simulink model "air_speed_control"  (R2016a)
settings: Solver=VariableStepAuto  StartTime=0.0  StopTime=10.0  RelTol=1e-6
model workspace (MAT data in the model file):
  A1 = 0.00125663706144
  A2 = 0.00105557513161
  L = 0.3
  M_huosai = 20
  P0 = 101300
  R = 287.1
  T1 = 293
  T2 = 293
  Ts = 293
  k = 1.4
undefined symbols (not defined in the file or in its folder): vd
settings Model: Creator=xlh  LastModifiedBy=xlh

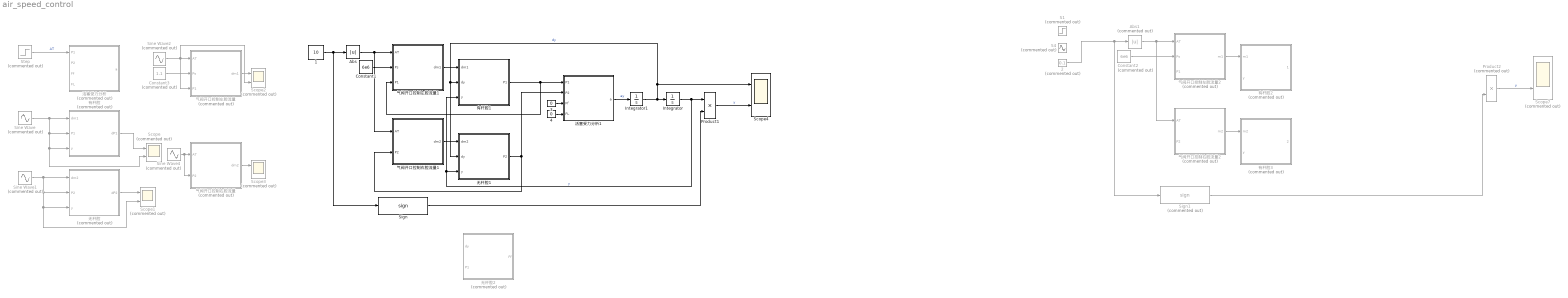
== system air_speed_control ==
  1 : Constant  Value=10
  2 : Constant  Commented=on  Value=0.1
  3 : Constant  Value=0
  4 : Constant  Value=0
  Abs : Abs
  Abs1 : Abs  Commented=on
  Constant1 : Constant  Value=6e6
  Constant2 : Constant  Commented=on  Value=6e6
  Constant3 : Constant  Commented=on  Value=1.1
  Integrator : Integrator
  Integrator1 : Integrator
  Product1 : Product
  Product2 : Product  Commented=on
  S1 : Step  Commented=on  SampleTime=0
  S4 : Sin  Commented=on  SampleTime=0
  Scope{,1..3,7} (5 alike) : Scope  Commented=on  NumInputPorts=2
  Scope4 : Scope  NumInputPorts=2
  Sign : Signum
  Sign1 : Signum  Commented=on
  Sine Wave{,1..2,4} (4 alike) : Sin  Commented=on  SampleTime=0
  Step : Step  Commented=on  SampleTime=0
  无杆腔 : Subsystem  Commented=on
  无杆腔1 : Subsystem
  无杆腔2 : Subsystem  Commented=on
  有杆腔 : Subsystem  Commented=on
  有杆腔1 : Subsystem
  有杆腔2 : Subsystem  Commented=on
  有杆腔3 : Subsystem  Commented=on
  气阀开口控制右腔流量 : Subsystem  Commented=on
  气阀开口控制右腔流量1 : Subsystem
  气阀开口控制右腔流量2 : Subsystem  Commented=on
  气阀开口控制左腔流量 : Subsystem  Commented=on
  气阀开口控制左腔流量1 : Subsystem
  气阀开口控制左腔流量2 : Subsystem  Commented=on
  活塞受力分析 : Subsystem  Commented=on
  活塞受力分析1 : Subsystem
  wires:
  Step/1 -> 活塞受力分析/1(P1)  "AT"
  Sine Wave/1 -> Scope/2, 有杆腔/3(y), 有杆腔/2(P1), 有杆腔/1(dm1)
  有杆腔/1(dP1) -> Scope/1
  Sine Wave1/1 -> Scope1/2, 无杆腔/3(y), 无杆腔/2(P2), 无杆腔/1(dm2)
  无杆腔/1(dP2) -> Scope1/1
  Constant3/1 -> 气阀开口控制左腔流量/2(Ps)
  Sine Wave2/1 -> 气阀开口控制左腔流量/3(P1), Scope2/2, 气阀开口控制左腔流量/1(AT)
  气阀开口控制左腔流量/1(dm1) -> Scope2/1
  Sine Wave4/1 -> 气阀开口控制右腔流量/2(P2), 气阀开口控制右腔流量/1(AT)
  气阀开口控制右腔流量/1(dm2) -> Scope3/1
  气阀开口控制左腔流量1/1(dm1) -> 有杆腔1/1(dm1)
  有杆腔1/1(P1) -> 气阀开口控制左腔流量1/3(P1), 活塞受力分析1/1(P1)
  活塞受力分析1/1(a) -> Integrator1/1  "ay"
  Integrator1/1 -> Integrator/1, 有杆腔1/2(dy), 无杆腔1/2(dy), Scope4/1  "dy"
  Constant1/1 -> 气阀开口控制左腔流量1/2(Ps)
  气阀开口控制右腔流量1/1(dm2) -> 无杆腔1/1(dm2)
  4/1 -> 活塞受力分析1/4(FL)
  无杆腔1/1(P2) -> 活塞受力分析1/2(P2), 气阀开口控制右腔流量1/2(P2)
  Integrator/1 -> 无杆腔1/3(y), 有杆腔1/3(y), Product1/1  "y"
  Product1/1 -> Scope4/2  "y"
  Sign/1 -> Product1/2
  1/1 -> Abs/1, Sign/1
  Abs/1 -> 气阀开口控制右腔流量1/1(AT), 气阀开口控制左腔流量1/1(AT)
  气阀开口控制左腔流量2/1(m1) -> 有杆腔2/1(m1)
  Constant2/1 -> 气阀开口控制左腔流量2/2(Ps)
  Product2/1 -> Scope7/2  "y"
  Sign1/1 -> Product2/2
  2/1 -> Abs1/1, Sign1/1
  Abs1/1 -> 气阀开口控制右腔流量2/1(AT), 气阀开口控制左腔流量2/1(AT)
  气阀开口控制右腔流量2/1(m2) -> 有杆腔3/1(m2)
  3/1 -> 活塞受力分析1/3(Ff)

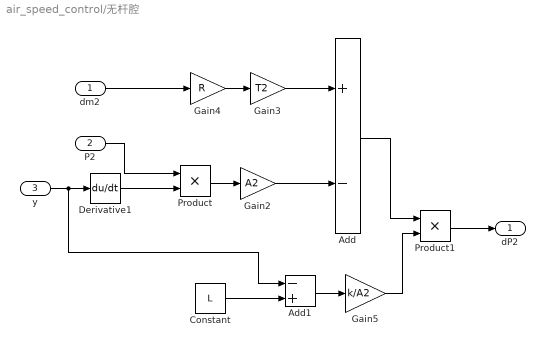
== system air_speed_control/无杆腔 ==
  dm2 : Inport
  P2 : Inport  Port=2
  y : Inport  Port=3
  Add : Sum  Inputs=+-
  Add1 : Sum  Inputs=-+
  Constant : Constant  Value=L
  Derivative1 : Derivative
  Gain2 : Gain  Gain=A2
  Gain3 : Gain  Gain=T2
  Gain4 : Gain  Gain=R
  Gain5 : Gain  Gain=k/A2
  Product : Product
  Product1 : Product
  dP2 : Outport
  wires:
  Gain5/1 -> Product1/2
  Add1/1 -> Gain5/1
  Constant/1 -> Add1/2
  Derivative1/1 -> Product/2
  y/1 -> Derivative1/1, Add1/1
  Gain3/1 -> Add/1
  dm2/1 -> Gain4/1
  Gain4/1 -> Gain3/1
  Gain2/1 -> Add/2
  Product/1 -> Gain2/1
  P2/1 -> Product/1
  Add/1 -> Product1/1
  Product1/1 -> dP2/1

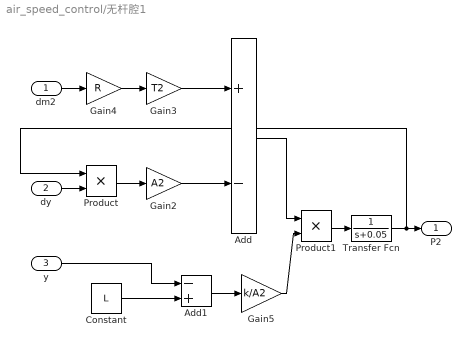
== system air_speed_control/无杆腔1 ==
  dm2 : Inport
  dy : Inport  Port=2
  y : Inport  Port=3
  Add : Sum  Inputs=+-
  Add1 : Sum  Inputs=-+
  Constant : Constant  Value=L
  Gain2 : Gain  Gain=A2
  Gain3 : Gain  Gain=T2
  Gain4 : Gain  Gain=R
  Gain5 : Gain  Gain=k/A2
  Product : Product
  Product1 : Product
  Transfer Fcn : TransferFcn  Denominator=[1 0.05]
  P2 : Outport
  wires:
  Product1/1 -> Transfer Fcn/1
  Add/1 -> Product1/1
  Transfer Fcn/1 -> Product/1, P2/1
  Product/1 -> Gain2/1
  Gain2/1 -> Add/2
  Gain4/1 -> Gain3/1
  dm2/1 -> Gain4/1
  Gain3/1 -> Add/1
  dy/1 -> Product/2
  Constant/1 -> Add1/2
  Add1/1 -> Gain5/1
  Gain5/1 -> Product1/2
  y/1 -> Add1/1

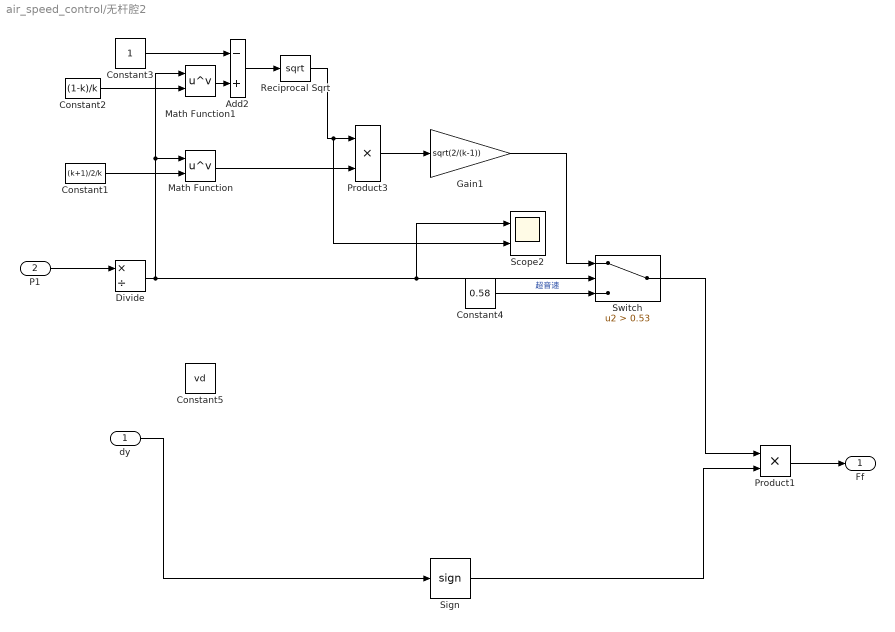
== system air_speed_control/无杆腔2 ==
  dy : Inport
  P1 : Inport  Port=2
  Add2 : Sum  Inputs=-+
  Constant1 : Constant  Value=(k+1)/2/k
  Constant2 : Constant  Value=(1-k)/k
  Constant3 : Constant
  Constant4 : Constant  Value=0.58
  Constant5 : Constant  Value=vd
  Divide : Product  Inputs=*/
  Gain1 : Gain  Gain=sqrt(2/(k-1))
  Math Function : Math  Operator=pow  SaturateOnIntegerOverflow=on
  Math Function1 : Math  Operator=pow  SaturateOnIntegerOverflow=on
  Product1 : Product
  Product3 : Product
  Reciprocal Sqrt : Sqrt  SaturateOnIntegerOverflow=on
  Scope2 : Scope  NumInputPorts=2
  Sign : Signum
  Switch : Switch  Criteria=u2 > Threshold  Threshold=0.53
  Ff : Outport
  wires:
  dy/1 -> Sign/1
  Product1/1 -> Ff/1
  Sign/1 -> Product1/2
  Constant4/1 -> Switch/3  "超音速"
  Gain1/1 -> Switch/1
  Product3/1 -> Gain1/1
  Reciprocal Sqrt/1 -> Product3/1, Scope2/2
  Add2/1 -> Reciprocal Sqrt/1
  Constant3/1 -> Add2/1
  Math Function1/1 -> Add2/2
  Constant2/1 -> Math Function1/2
  Math Function/1 -> Product3/2
  Constant1/1 -> Math Function/2
  Divide/1 -> Switch/2, Scope2/1, Math Function/1, Math Function1/1
  P1/1 -> Divide/1
  Switch/1 -> Product1/1

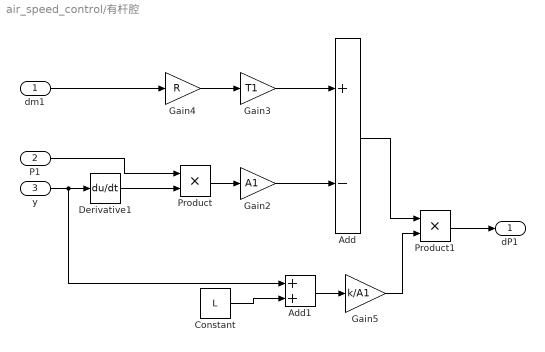
== system air_speed_control/有杆腔 ==
  dm1 : Inport
  P1 : Inport  Port=2
  y : Inport  Port=3
  Add : Sum  Inputs=+-
  Add1 : Sum
  Constant : Constant  Value=L
  Derivative1 : Derivative
  Gain2 : Gain  Gain=A1
  Gain3 : Gain  Gain=T1
  Gain4 : Gain  Gain=R
  Gain5 : Gain  Gain=k/A1
  Product : Product
  Product1 : Product
  dP1 : Outport
  wires:
  Product1/1 -> dP1/1
  Add/1 -> Product1/1
  P1/1 -> Product/1
  Product/1 -> Gain2/1
  Gain2/1 -> Add/2
  Gain4/1 -> Gain3/1
  dm1/1 -> Gain4/1
  Gain3/1 -> Add/1
  y/1 -> Add1/1, Derivative1/1
  Derivative1/1 -> Product/2
  Constant/1 -> Add1/2
  Add1/1 -> Gain5/1
  Gain5/1 -> Product1/2

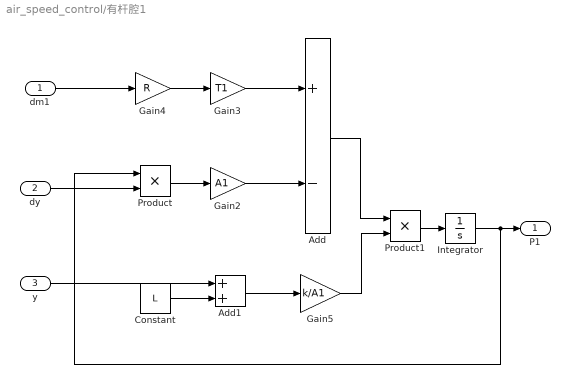
== system air_speed_control/有杆腔1 ==
  dm1 : Inport
  dy : Inport  Port=2
  y : Inport  Port=3
  Add : Sum  Inputs=+-
  Add1 : Sum
  Constant : Constant  Value=L
  Gain2 : Gain  Gain=A1
  Gain3 : Gain  Gain=T1
  Gain4 : Gain  Gain=R
  Gain5 : Gain  Gain=k/A1
  Integrator : Integrator
  Product : Product
  Product1 : Product
  P1 : Outport
  wires:
  Gain5/1 -> Product1/2
  Add1/1 -> Gain5/1
  Constant/1 -> Add1/2
  dy/1 -> Product/2
  Gain3/1 -> Add/1
  dm1/1 -> Gain4/1
  Gain4/1 -> Gain3/1
  Gain2/1 -> Add/2
  Product/1 -> Gain2/1
  Add/1 -> Product1/1
  Product1/1 -> Integrator/1
  Integrator/1 -> Product/1, P1/1
  y/1 -> Add1/1

== system air_speed_control/有杆腔2 ==
  m1 : Inport
  y : Inport  Port=2
  Add1 : Sum
  Constant : Constant  Value=L
  Gain1 : Gain  Gain=1+k
  Gain5 : Gain  Gain=k*R*T1
  Product1 : Product
  1 : Outport
  wires:
  Gain5/1 -> Product1/2
  Add1/1 -> Gain5/1
  Constant/1 -> Add1/2
  Product1/1 -> 1/1
  y/1 -> Gain1/1
  Gain1/1 -> Add1/1
  m1/1 -> Product1/1

== system air_speed_control/有杆腔3 ==
  m2 : Inport
  y : Inport  Port=2
  Add1 : Sum  Inputs=-+
  Constant : Constant  Value=L
  Gain1 : Gain  Gain=1+k
  Gain5 : Gain  Gain=k*R*T2
  Product1 : Product
  2 : Outport
  wires:
  m2/1 -> Product1/1
  Gain1/1 -> Add1/1
  y/1 -> Gain1/1
  Product1/1 -> 2/1
  Constant/1 -> Add1/2
  Add1/1 -> Gain5/1
  Gain5/1 -> Product1/2

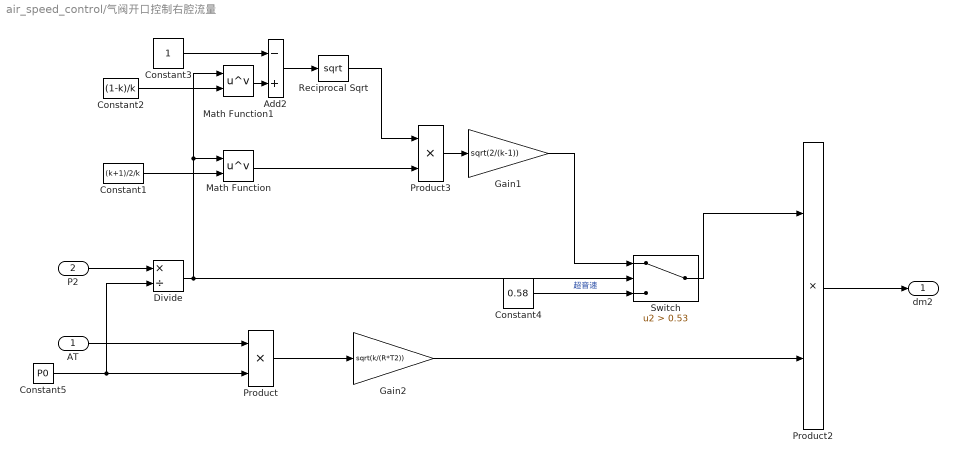
== system air_speed_control/气阀开口控制右腔流量 ==
  AT : Inport
  P2 : Inport  Port=2
  Add2 : Sum  Inputs=-+
  Constant1 : Constant  Value=(k+1)/2/k
  Constant2 : Constant  Value=(1-k)/k
  Constant3 : Constant
  Constant4 : Constant  Value=0.58
  Constant5 : Constant  Value=P0
  Divide : Product  Inputs=*/
  Gain1 : Gain  Gain=sqrt(2/(k-1))
  Gain2 : Gain  Gain=sqrt(k/(R*T2))
  Math Function : Math  Operator=pow  SaturateOnIntegerOverflow=on
  Math Function1 : Math  Operator=pow  SaturateOnIntegerOverflow=on
  Product : Product
  Product2 : Product
  Product3 : Product
  Reciprocal Sqrt : Sqrt  SaturateOnIntegerOverflow=on
  Switch : Switch  Criteria=u2 > Threshold  Threshold=0.53
  dm2 : Outport
  wires:
  Product2/1 -> dm2/1
  Constant4/1 -> Switch/3  "超音速"
  Gain1/1 -> Switch/1
  Product3/1 -> Gain1/1
  Reciprocal Sqrt/1 -> Product3/1
  Add2/1 -> Reciprocal Sqrt/1
  Constant3/1 -> Add2/1
  Math Function1/1 -> Add2/2
  Constant2/1 -> Math Function1/2
  Math Function/1 -> Product3/2
  Constant1/1 -> Math Function/2
  Divide/1 -> Switch/2, Math Function/1, Math Function1/1
  P2/1 -> Divide/1
  Switch/1 -> Product2/1
  AT/1 -> Product/1
  Product/1 -> Gain2/1
  Gain2/1 -> Product2/2
  Constant5/1 -> Product/2, Divide/2

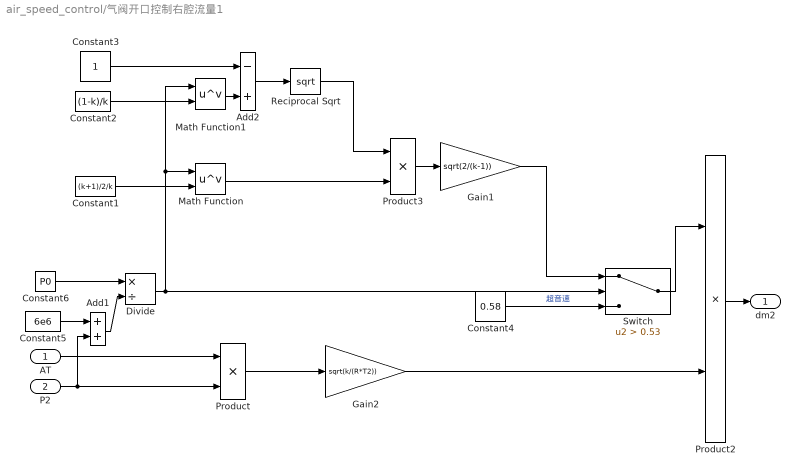
== system air_speed_control/气阀开口控制右腔流量1 ==
  AT : Inport
  P2 : Inport  Port=2
  Add1 : Sum
  Add2 : Sum  Inputs=-+
  Constant1 : Constant  Value=(k+1)/2/k
  Constant2 : Constant  Value=(1-k)/k
  Constant3 : Constant
  Constant4 : Constant  Value=0.58
  Constant5 : Constant  Value=6e6
  Constant6 : Constant  Value=P0
  Divide : Product  Inputs=*/
  Gain1 : Gain  Gain=sqrt(2/(k-1))
  Gain2 : Gain  Gain=sqrt(k/(R*T2))
  Math Function : Math  Operator=pow  SaturateOnIntegerOverflow=on
  Math Function1 : Math  Operator=pow  SaturateOnIntegerOverflow=on
  Product : Product
  Product2 : Product
  Product3 : Product
  Reciprocal Sqrt : Sqrt  SaturateOnIntegerOverflow=on
  Switch : Switch  Criteria=u2 > Threshold  Threshold=0.53
  dm2 : Outport
  wires:
  P2/1 -> Add1/2, Product/2
  Gain2/1 -> Product2/2
  Product/1 -> Gain2/1
  AT/1 -> Product/1
  Switch/1 -> Product2/1
  Divide/1 -> Math Function1/1, Math Function/1, Switch/2
  Constant1/1 -> Math Function/2
  Math Function/1 -> Product3/2
  Constant2/1 -> Math Function1/2
  Math Function1/1 -> Add2/2
  Constant3/1 -> Add2/1
  Add2/1 -> Reciprocal Sqrt/1
  Reciprocal Sqrt/1 -> Product3/1
  Product3/1 -> Gain1/1
  Gain1/1 -> Switch/1
  Constant4/1 -> Switch/3  "超音速"
  Product2/1 -> dm2/1
  Constant6/1 -> Divide/1
  Constant5/1 -> Add1/1
  Add1/1 -> Divide/2

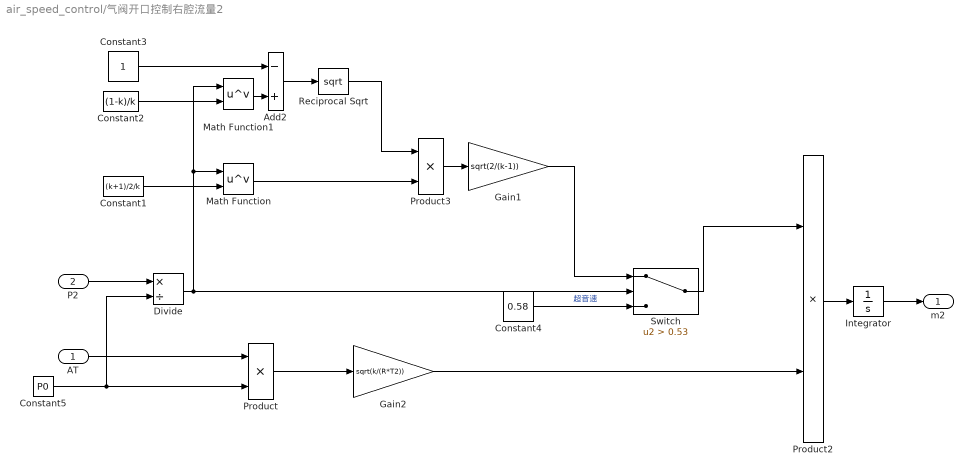
== system air_speed_control/气阀开口控制右腔流量2 ==
  AT : Inport
  P2 : Inport  Port=2
  Add2 : Sum  Inputs=-+
  Constant1 : Constant  Value=(k+1)/2/k
  Constant2 : Constant  Value=(1-k)/k
  Constant3 : Constant
  Constant4 : Constant  Value=0.58
  Constant5 : Constant  Value=P0
  Divide : Product  Inputs=*/
  Gain1 : Gain  Gain=sqrt(2/(k-1))
  Gain2 : Gain  Gain=sqrt(k/(R*T2))
  Integrator : Integrator
  Math Function : Math  Operator=pow  SaturateOnIntegerOverflow=on
  Math Function1 : Math  Operator=pow  SaturateOnIntegerOverflow=on
  Product : Product
  Product2 : Product
  Product3 : Product
  Reciprocal Sqrt : Sqrt  SaturateOnIntegerOverflow=on
  Switch : Switch  Criteria=u2 > Threshold  Threshold=0.53
  m2 : Outport
  wires:
  Constant5/1 -> Divide/2, Product/2
  Gain2/1 -> Product2/2
  Product/1 -> Gain2/1
  AT/1 -> Product/1
  Switch/1 -> Product2/1
  P2/1 -> Divide/1
  Divide/1 -> Math Function1/1, Math Function/1, Switch/2
  Constant1/1 -> Math Function/2
  Math Function/1 -> Product3/2
  Constant2/1 -> Math Function1/2
  Math Function1/1 -> Add2/2
  Constant3/1 -> Add2/1
  Add2/1 -> Reciprocal Sqrt/1
  Reciprocal Sqrt/1 -> Product3/1
  Product3/1 -> Gain1/1
  Gain1/1 -> Switch/1
  Constant4/1 -> Switch/3  "超音速"
  Product2/1 -> Integrator/1
  Integrator/1 -> m2/1

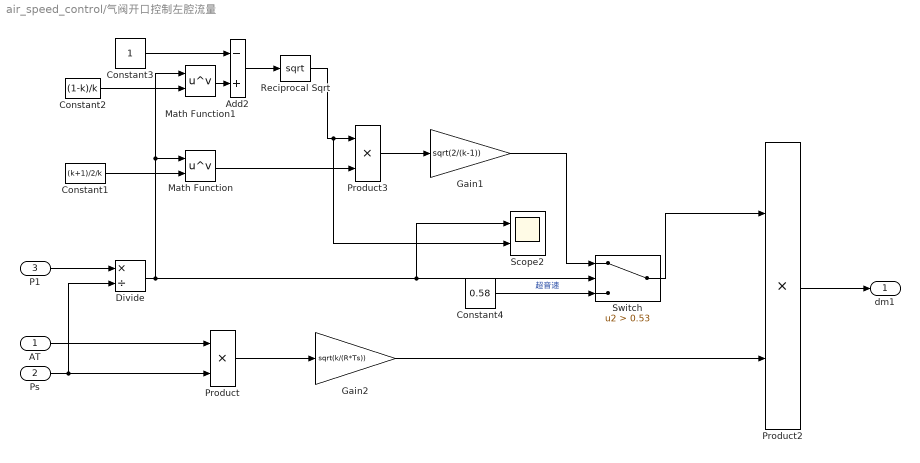
== system air_speed_control/气阀开口控制左腔流量 ==
  AT : Inport
  Ps : Inport  Port=2
  P1 : Inport  Port=3
  Add2 : Sum  Inputs=-+
  Constant1 : Constant  Value=(k+1)/2/k
  Constant2 : Constant  Value=(1-k)/k
  Constant3 : Constant
  Constant4 : Constant  Value=0.58
  Divide : Product  Inputs=*/
  Gain1 : Gain  Gain=sqrt(2/(k-1))
  Gain2 : Gain  Gain=sqrt(k/(R*Ts))
  Math Function : Math  Operator=pow  SaturateOnIntegerOverflow=on
  Math Function1 : Math  Operator=pow  SaturateOnIntegerOverflow=on
  Product : Product
  Product2 : Product
  Product3 : Product
  Reciprocal Sqrt : Sqrt  SaturateOnIntegerOverflow=on
  Scope2 : Scope  NumInputPorts=2
  Switch : Switch  Criteria=u2 > Threshold  Threshold=0.53
  dm1 : Outport
  wires:
  Ps/1 -> Divide/2, Product/2
  Gain2/1 -> Product2/2
  Product/1 -> Gain2/1
  AT/1 -> Product/1
  Switch/1 -> Product2/1
  P1/1 -> Divide/1
  Divide/1 -> Math Function1/1, Math Function/1, Scope2/1, Switch/2
  Constant1/1 -> Math Function/2
  Math Function/1 -> Product3/2
  Constant2/1 -> Math Function1/2
  Math Function1/1 -> Add2/2
  Constant3/1 -> Add2/1
  Add2/1 -> Reciprocal Sqrt/1
  Reciprocal Sqrt/1 -> Scope2/2, Product3/1
  Product3/1 -> Gain1/1
  Gain1/1 -> Switch/1
  Constant4/1 -> Switch/3  "超音速"
  Product2/1 -> dm1/1

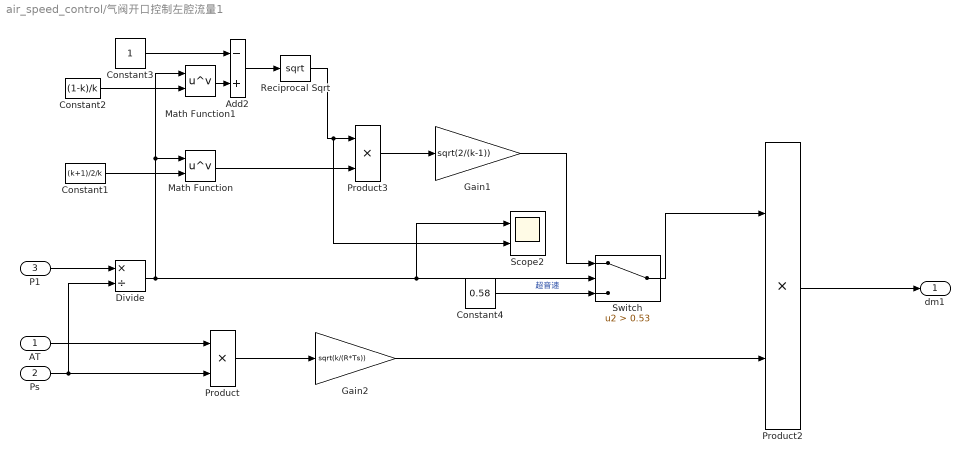
== system air_speed_control/气阀开口控制左腔流量1 ==
  AT : Inport
  Ps : Inport  Port=2
  P1 : Inport  Port=3
  Add2 : Sum  Inputs=-+
  Constant1 : Constant  Value=(k+1)/2/k
  Constant2 : Constant  Value=(1-k)/k
  Constant3 : Constant
  Constant4 : Constant  Value=0.58
  Divide : Product  Inputs=*/
  Gain1 : Gain  Gain=sqrt(2/(k-1))
  Gain2 : Gain  Gain=sqrt(k/(R*Ts))
  Math Function : Math  Operator=pow  SaturateOnIntegerOverflow=on
  Math Function1 : Math  Operator=pow  OutputSignalType=real  SaturateOnIntegerOverflow=on
  Product : Product
  Product2 : Product
  Product3 : Product
  Reciprocal Sqrt : Sqrt  OutputSignalType=real  SaturateOnIntegerOverflow=on
  Scope2 : Scope  NumInputPorts=2
  Switch : Switch  Criteria=u2 > Threshold  Threshold=0.53
  dm1 : Outport
  wires:
  Product2/1 -> dm1/1
  Constant4/1 -> Switch/3  "超音速"
  Gain1/1 -> Switch/1
  Product3/1 -> Gain1/1
  Reciprocal Sqrt/1 -> Product3/1, Scope2/2
  Add2/1 -> Reciprocal Sqrt/1
  Constant3/1 -> Add2/1
  Math Function1/1 -> Add2/2
  Constant2/1 -> Math Function1/2
  Math Function/1 -> Product3/2
  Constant1/1 -> Math Function/2
  Divide/1 -> Switch/2, Scope2/1, Math Function/1, Math Function1/1
  P1/1 -> Divide/1
  Switch/1 -> Product2/1
  AT/1 -> Product/1
  Product/1 -> Gain2/1
  Gain2/1 -> Product2/2
  Ps/1 -> Product/2, Divide/2

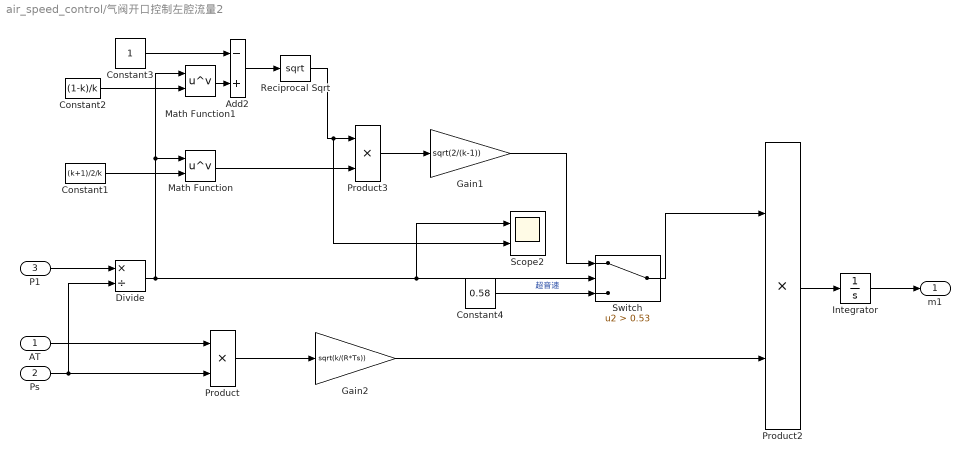
== system air_speed_control/气阀开口控制左腔流量2 ==
  AT : Inport
  Ps : Inport  Port=2
  P1 : Inport  Port=3
  Add2 : Sum  Inputs=-+
  Constant1 : Constant  Value=(k+1)/2/k
  Constant2 : Constant  Value=(1-k)/k
  Constant3 : Constant
  Constant4 : Constant  Value=0.58
  Divide : Product  Inputs=*/
  Gain1 : Gain  Gain=sqrt(2/(k-1))
  Gain2 : Gain  Gain=sqrt(k/(R*Ts))
  Integrator : Integrator
  Math Function : Math  Operator=pow  SaturateOnIntegerOverflow=on
  Math Function1 : Math  Operator=pow  SaturateOnIntegerOverflow=on
  Product : Product
  Product2 : Product
  Product3 : Product
  Reciprocal Sqrt : Sqrt  SaturateOnIntegerOverflow=on
  Scope2 : Scope  NumInputPorts=2
  Switch : Switch  Criteria=u2 > Threshold  Threshold=0.53
  m1 : Outport
  wires:
  Product2/1 -> Integrator/1
  Constant4/1 -> Switch/3  "超音速"
  Gain1/1 -> Switch/1
  Product3/1 -> Gain1/1
  Reciprocal Sqrt/1 -> Product3/1, Scope2/2
  Add2/1 -> Reciprocal Sqrt/1
  Constant3/1 -> Add2/1
  Math Function1/1 -> Add2/2
  Constant2/1 -> Math Function1/2
  Math Function/1 -> Product3/2
  Constant1/1 -> Math Function/2
  Divide/1 -> Switch/2, Scope2/1, Math Function/1, Math Function1/1
  P1/1 -> Divide/1
  Switch/1 -> Product2/1
  AT/1 -> Product/1
  Product/1 -> Gain2/1
  Gain2/1 -> Product2/2
  Ps/1 -> Product/2, Divide/2
  Integrator/1 -> m1/1

== system air_speed_control/活塞受力分析 ==
  note: P2
  P1 : Inport
  P2 : Inport  Port=2
  Ff : Inport  Port=3
  FL : Inport  Port=4
  Add : Sum  Inputs=+---
  Gain1 : Gain  Gain=M_huosai
  Gain2 : Gain  Gain=A1
  Gain3 : Gain  Gain=A2
  a : Outport
  wires:
  P1/1 -> Gain2/1  "P1"
  P2/1 -> Gain3/1
  Ff/1 -> Add/3  "Ff"
  FL/1 -> Add/4  "FL"
  Gain2/1 -> Add/1
  Gain3/1 -> Add/2
  Add/1 -> Gain1/1
  Gain1/1 -> a/1  "a"

== system air_speed_control/活塞受力分析1 ==
  note: P2
  P1 : Inport
  P2 : Inport  Port=2
  Ff : Inport  Port=3
  FL : Inport  Port=4
  Add : Sum  Inputs=+---
  Gain1 : Gain  Gain=1/M_huosai
  Gain2 : Gain  Gain=A1
  Gain3 : Gain  Gain=A2
  a : Outport
  wires:
  Gain1/1 -> a/1  "a"
  Add/1 -> Gain1/1
  Gain3/1 -> Add/2
  Gain2/1 -> Add/1
  FL/1 -> Add/4  "FL"
  Ff/1 -> Add/3  "Ff"
  P2/1 -> Gain3/1
  P1/1 -> Gain2/1  "P1"
